simulink model "stp1_3sym"  (R2022b)
settings: Solver=VariableStepAuto  StartTime=0.0  StopTime=12  RelTol=1e-3
values from neighbouring files (symbols this model uses):
  K = inv(M'*M + lambda*eye(Nu)) * M'    [dmc.m]    (also in dpid.m = 7.7; gpc.m; stp1.m = acker(A, B, [s s s]))
  x1_0 = 2    [stp1.m]
  x2_0 = 1    [stp1.m]
  x3_0 = -1    [stp1.m]
settings Model: Creator=zalew  LastModifiedBy=zalew

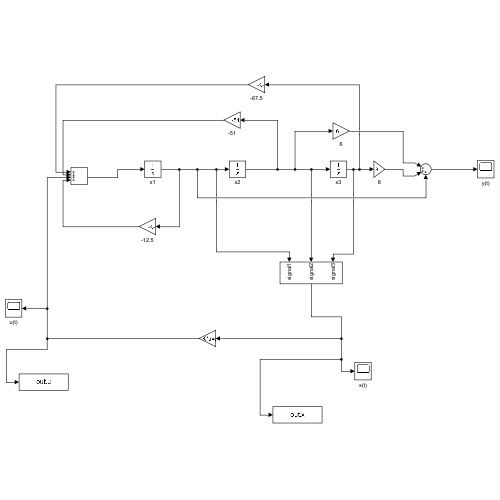
[thumbnail: Simulink's stored preview of the top-level diagram]
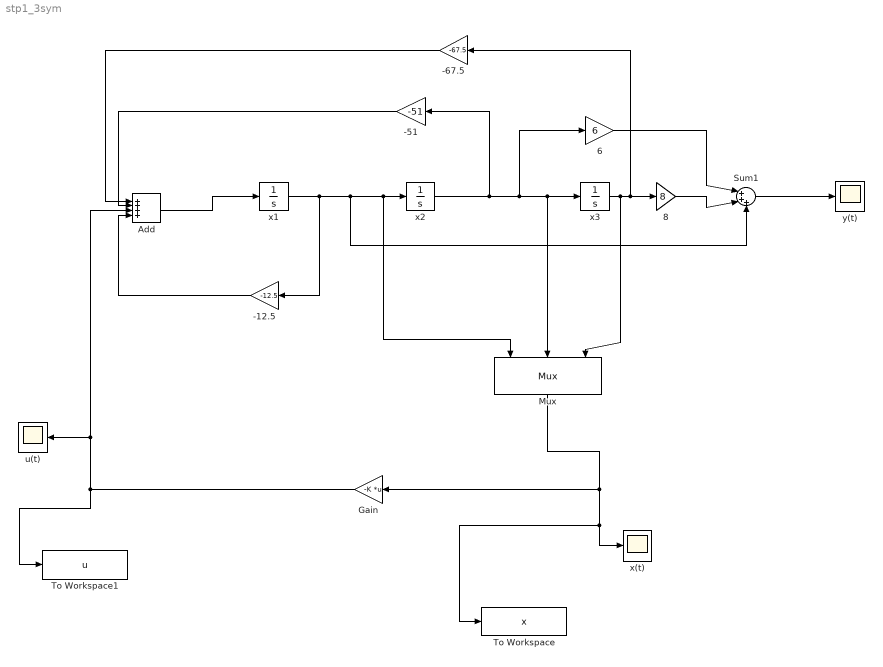
== system stp1_3sym ==
  -12.5 : Gain  Gain=-12.5
  -51 : Gain  Gain=-51
  -67.5 : Gain  Gain=-67.5
  6 : Gain  Gain=6
  8 : Gain  Gain=8
  Add : Sum  Inputs=++++
  Gain : Gain  Gain=-K  Multiplication=Matrix(K*u) (u vector)
  Mux : Mux  Inputs=3
      settings: DisplayOption=signals
  Sum1 : Sum  Inputs=|+++
  To Workspace : ToWorkspace  VariableName=x  SaveFormat=Structure With Time  SampleTime=-1
  To Workspace1 : ToWorkspace  VariableName=u  SaveFormat=Structure With Time  SampleTime=-1
  u(t) : Scope
  x(t) : Scope
  x1 : Integrator  InitialCondition=x1_0
  x2 : Integrator  InitialCondition=x2_0
  x3 : Integrator  InitialCondition=x3_0
  y(t) : Scope
  wires:
  Mux/1 -> To Workspace/1, x(t)/1, Gain/1
  x1/1 -> -12.5/1, Mux/1, x2/1, Sum1/3
  Gain/1 -> u(t)/1, Add/3, To Workspace1/1
  8/1 -> Sum1/2
  x2/1 -> x3/1, Mux/2, 6/1, -51/1
  x3/1 -> Mux/3, -67.5/1, 8/1
  Add/1 -> x1/1
  -67.5/1 -> Add/1
  -12.5/1 -> Add/4
  6/1 -> Sum1/1
  -51/1 -> Add/2
  Sum1/1 -> y(t)/1
